simulink model "parameter_estimation_hardware"  (R2019a)
settings: Solver=ode1  StartTime=0.0  StopTime=inf  FixedStep=0.001  RelTol=1e-3
undefined symbols (not defined in the file): A0, af, bf, bhat0, HIL, k, Kt, lambda, mhat0, Nenc, omega, phi, qc_get_step_size, R, r_enc, rg, rm, T, Vmax
libraries: quarc_library x3
settings Model: SimulationMode=external  ExtModeTrigDuration=5000  Creator=johnchiasson  LastModifiedBy=NardosAshenafi
settings SolverCC: PositivePriorityOrder=on
settings DataIOCC: LimitDataPoints=on  SaveFormat=Array  ReturnWorkspaceOutputs=off
settings OptimizationCC: LifeSpan=inf
settings DebuggingCC: SFUnexpectedBacktrackingDiag=warning  SFNoUnconditionalDefaultTransitionDiag=warning  SFExecutionAtInitializationDiag=none  ArithmeticOperatorsInVariantConditions=warning
settings HardwareCC: ProdBitPerPointer=32  ProdBitPerSizeT=32  ProdBitPerPtrDiffT=32  ProdLargestAtomicFloat=None  ProdIntDivRoundTo=Undefined  ProdEndianess=Unspecified  ProdWordSize=32  ProdHWDeviceType=32-bit Generic
settings ModelReferenceCC: PropagateSignalLabelsOutOfModel=off
settings SFSimCC: SimUseLocalCustomCode=off
settings RTWCC: SystemTargetFile=quarc_win64.tlc  TemplateMakefile=quarc_default_tmf  Description=QUARC Win64 Target  RTWUseLocalCustomCode=off
settings CodeAppCC: StateflowObjectComments=on
settings STFCustomTargetCC: TargetPreCompLibLocation=C:\PROGRA~3\QUARC\lib\2019a\win64\release  ConcurrentExecutionCompliant=on  SystemTargetFile=quarc_win64.tlc
settings GRTTargetCC: TargetPreCompLibLocation=C:\PROGRA~3\QUARC\lib\2019a\win64\release  TargetLangStandard=C89/C90 (ANSI)  ParMdlRefBuildCompliant=off  CompOptLevelCompliant=off  CombineOutputUpdateFcns=off  MatFileLogging=off  CPPClassGenCompliant=off  GRTInterface=on  UseToolchainInfoCompliant=off  ExtMode=on  ExtModeMexFile=quarc_comm
settings ConfigComp: CovMetricSettings=dw  CovSaveCumulativeToWorkspaceVar=on  CovSaveSingleToWorkspaceVar=on  CovExternalEMLEnable=off

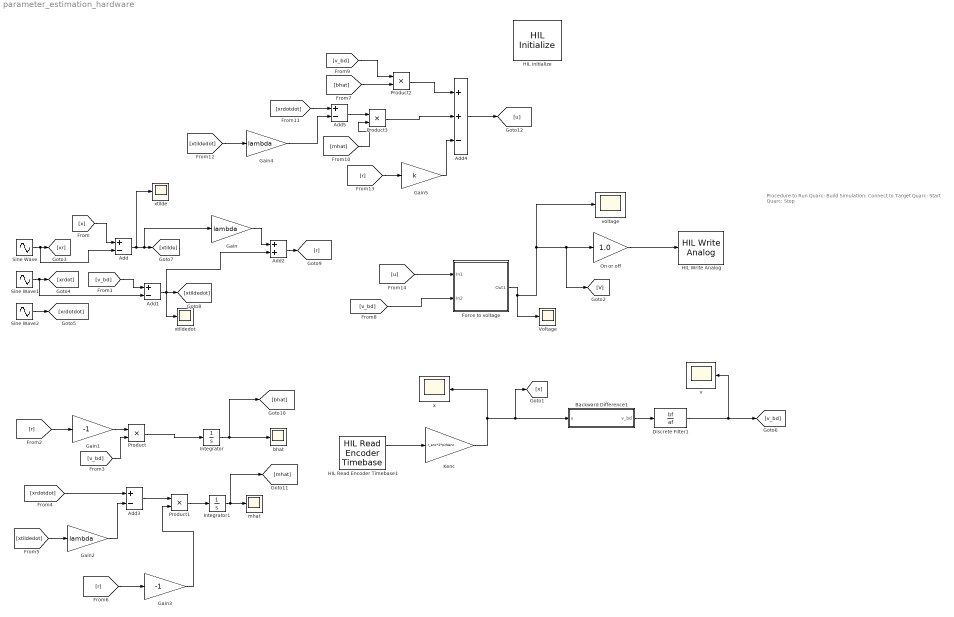
== system parameter_estimation_hardware ==
  note: Procedure to Run
      |
      | Quarc: Build
      | Simulation: Connect to Target
      | Quarc: Start
      | Quarc: Stop
  Add{,1,3,5} (4 alike) : Sum  Inputs=+-
  Add2 : Sum
  Add4 : Sum  Inputs=++-
  Backward Difference1 : Subsystem
  Discrete Filter1 : DiscreteFilter  Numerator=bf  Denominator=af
  Force to voltage : Subsystem
  Gain : Gain  Gain=lambda
  Gain1 : Gain  Gain=-1
  Gain2 : Gain  Gain=lambda
  Gain3 : Gain  Gain=-1
  Gain4 : Gain  Gain=lambda
  Gain5 : Gain  Gain=k
  HIL Initialize : quarc_library/Data Acquisition/Generic/Configuration/HIL Initialize  Priority=-99  object_name=HIL-1  board_type=q2_usb  board_number=0  board_options=d0=digital;d1=digital;led=auto;update_rate=normal;decimation=1  exclusive=off  active=off  hardware_clocks=[0]  clock_modes=[]  initial_clock_frequencies=[]  set_clock_params_at_start=off  set_clock_params_at_switch_in=off  set_clock_frequencies_at_start=off  set_clock_frequencies_at_switch_in=off  analog_input_channels=[0:1]  analog_input_configurations=[]  analog_input_maximums=10  analog_input_minimums=-10  set_analog_input_params_at_start=on  set_analog_input_params_at_switch_in=off  analog_output_channels=[0:1]  analog_output_maximums=10  analog_output_minimums=-10  initial_analog_outputs=[0]  final_analog_outputs=[0]  watchdog_analog_outputs=0  set_analog_output_params_at_start=on  set_analog_output_params_at_switch_in=off  set_analog_outputs_at_start=on  set_analog_outputs_at_switch_in=off  set_analog_outputs_at_terminate=on  set_analog_outputs_at_switch_out=off  set_analog_outputs_on_watchdog=off  digital_input_channels=[]  digital_output_channels=[]  digital_output_configuration=[]  initial_digital_outputs=[1]  final_digital_outputs=[1]  watchdog_digital_outputs=[1]  set_digital_output_params_at_start=off  set_digital_output_params_at_switch_in=off  set_digital_outputs_at_start=on  set_digital_outputs_at_switch_in=off  set_digital_outputs_at_terminate=on  set_digital_outputs_at_switch_out=off  set_digital_outputs_on_watchdog=off  encoder_channels=[0:1]  quadrature=[4]  encoder_filter_frequency=[]  initial_encoder_counts=[0]  set_encoder_params_at_start=on  set_encoder_params_at_switch_in=off  set_encoder_counts_at_start=on  set_encoder_counts_at_switch_in=off  pwm_channels=[]  pwm_modes=[0]  pwm_frequency=1/0.020  pwm_configuration=[]  pwm_alignment=[]  pwm_polarity=[]  pwm_leading_deadband=[]  pwm_trailing_deadband=[]  initial_pwm_outputs=[0]  final_pwm_outputs=[0]  watchdog_pwm_outputs=[0]  set_pwm_params_at_start=on  set_pwm_params_at_switch_in=off  set_pwm_outputs_at_start=on  set_pwm_outputs_at_switch_in=off  set_pwm_outputs_at_terminate=on  set_pwm_outputs_at_switch_out=off  set_pwm_outputs_on_watchdog=off  other_output_channels=[]  initial_other_outputs=[]  final_other_outputs=[]  watchdog_other_outputs=[]  set_other_outputs_at_start=off  set_other_outputs_at_switch_in=off  set_other_outputs_at_terminate=off  set_other_outputs_at_switch_out=off  set_other_outputs_on_watchdog=off
  HIL Read Encoder Timebase1 : quarc_library/Data Acquisition/Generic/Timebases/HIL Read Encoder Timebase  object_name=HIL-1  clock=0  channels=[0:1]  samples_in_buffer=max(ceil(1/qc_get_step_size), 1)  active=on  vector_output=off  data_type_mode=Inherit via back propagation  data_type=double
  HIL Write Analog : quarc_library/Data Acquisition/Generic/Immediate I//O/HIL Write Analog  object_name=HIL-1  channels=0  sample_time=-1  active=off  vector_input=off
  Integrator : Integrator  InitialCondition=bhat0
  Integrator1 : Integrator  InitialCondition=mhat0
  Kenc : Gain  Gain=r_enc*2*pi/Nenc
  On or off : Gain  Gain=1.0
  Product{,1..3} (4 alike) : Product
  Sine Wave : Sin  Amplitude=A0  Frequency=omega  Phase=phi  SampleTime=0
  Sine Wave1 : Sin  Amplitude=A0*omega  Frequency=omega  Phase=phi + pi/2  SampleTime=0
  Sine Wave2 : Sin  Amplitude=-A0*omega*omega  Frequency=omega  Phase=phi  SampleTime=0
  Voltage : Scope
  bhat : Scope
  mhat : Scope
  v : Scope
  voltage : Scope
  x : Scope
  xtilde : Scope
  xtildedot : Scope
  wires:
  Add4/1 -> [u]
  Gain/1 -> Add2/1
  Integrator/1 -> [bhat], bhat/1
  Force to voltage/1(Out1) -> Voltage/1, On or off/1, [V], voltage/1
  Gain4/1 -> Add5/2
  Product1/1 -> Integrator1/1
  [v_bd] -> Add1/1
  Add5/1 -> Product3/1
  Add2/1 -> [r]
  [x] -> Add/1
  [mhat] -> Product3/2
  Add/1 -> xtilde/1, Gain/1, [xtilde]
  Product3/1 -> Add4/2
  Product2/1 -> Add4/1
  [xrdotdot] -> Add5/1
  [r] -> Gain3/1
  HIL Read Encoder Timebase1/1 -> Kenc/1
  Gain1/1 -> Product/1
  Gain3/1 -> Product1/2
  [xtildedot] -> Gain4/1
  [v_bd] -> Product2/1
  [bhat] -> Product2/2
  [r] -> Gain1/1
  [r] -> Gain5/1
  Sine Wave/1 -> Add/2, [xr]
  Backward Difference1/1(v_bd) -> Discrete Filter1/1
  Discrete Filter1/1 -> v/1, [v_bd]
  Add1/1 -> xtildedot/1, Add2/2, [xtildedot]
  Add3/1 -> Product1/1
  Gain2/1 -> Add3/2
  Gain5/1 -> Add4/3
  [u] -> Force to voltage/1(In1)
  [xrdotdot] -> Add3/1
  Sine Wave2/1 -> [xrdotdot]
  Product/1 -> Integrator/1
  Kenc/1 -> Backward Difference1/1(x), [x], x/1
  Sine Wave1/1 -> Add1/2, [xrdot]
  [v_bd] -> Product/2
  On or off/1 -> HIL Write Analog/1
  Integrator1/1 -> [mhat], mhat/1
  [xtildedot] -> Gain2/1
  [v_bd] -> Force to voltage/2(In2)

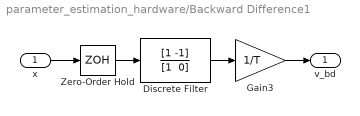
== system parameter_estimation_hardware/Backward Difference1 ==
  x : Inport
  Discrete Filter : DiscreteFilter  Numerator=[1 -1]  Denominator="[1  0]"
  Gain3 : Gain  Gain=1/T  SaturateOnIntegerOverflow=on  OutDataTypeStr=Inherit: Same as input  ParamDataTypeStr=Inherit: Same as input
  Zero-Order Hold : ZeroOrderHold  SampleTime=T
  v_bd : Outport
  wires:
  Discrete Filter/1 -> Gain3/1
  Gain3/1 -> v_bd/1
  Zero-Order Hold/1 -> Discrete Filter/1
  x/1 -> Zero-Order Hold/1

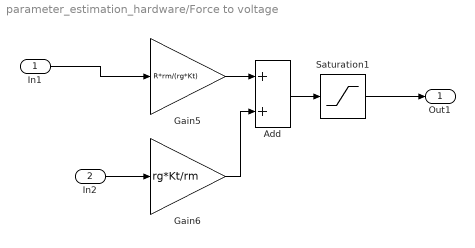
== system parameter_estimation_hardware/Force to voltage ==
  In1 : Inport
  In2 : Inport  Port=2
  Add : Sum
  Gain5 : Gain  Gain=R*rm/(rg*Kt)  SaturateOnIntegerOverflow=on  OutDataTypeStr=Inherit: Same as input  ParamDataTypeStr=Inherit: Same as input
  Gain6 : Gain  Gain=rg*Kt/rm  SaturateOnIntegerOverflow=on  OutDataTypeStr=Inherit: Same as input  ParamDataTypeStr=Inherit: Same as input
  Saturation1 : Saturate  UpperLimit=Vmax  LowerLimit=-Vmax
  Out1 : Outport  VectorParamsAs1DForOutWhenUnconnected=on
  wires:
  Add/1 -> Saturation1/1
  Gain5/1 -> Add/1
  Saturation1/1 -> Out1/1
  In1/1 -> Gain5/1
  Gain6/1 -> Add/2
  In2/1 -> Gain6/1
